simulink model "wlan_mac_hw"  (Simulink 7.8)
settings: Solver=ode45  StartTime=0.0  StopTime=200  RelTol=1e-3
PostLoadFcn:
  | wlan_mac_hw_init
InitFcn:
  | wlan_mac_hw_init
StartFcn:
  | wlan_mac_hw_init
values from neighbouring files (symbols this model uses):
  NB_CNTR_NAV = ceil(log2(MAX_NAV * 160))    [wlan_mac_hw_init.m]
  ticks_per_usec = 10    [wlan_mac_hw_init.m]
undefined symbols (not defined in the file or in its folder): gcbh, xlBlockLoadCallback, xlGetNormalizedPeriod
libraries: xbsIndex_r4 x788, xbsEDKLib_r4 x1
(part 4 of 6)

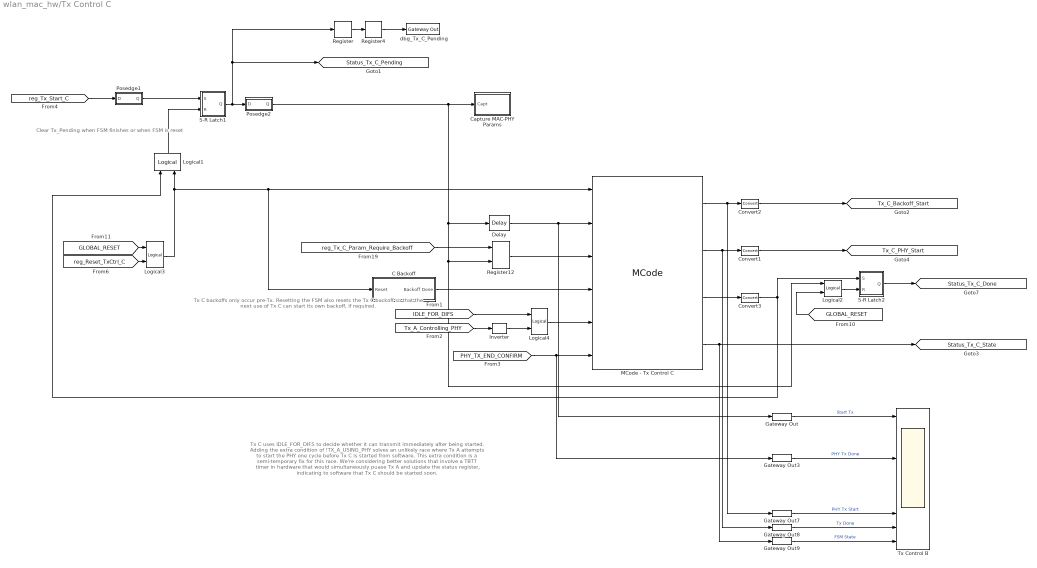
== system wlan_mac_hw/Tx Control C ==
  note: Clear Tx_Pending when FSM finishes
      | or when FSM is reset
  note: Tx C backoffs only occur pre-Tx. Resetting
      | the FSM also resets the Tx C backoff so that
      | the next use of Tx C can start its own backoff,
      | if required.
  note: Tx C uses IDLE_FOR_DIFS to decide whether it can
      | transmit immediately after being started. Adding the
      | extra condition of !TX_A_USING_PHY solves an unlikely
      | race where Tx A attempts to start the PHY one cycle
      | before Tx C is started from software.
      |
      | This extra condition is a semi-temporary fix for this race. We're
      | considering better solutions that involve a TBTT timer in
      | hardware that would simultaneously puase Tx A and update
      | the status register, indicating to software that Tx C should be
      | started soon.
  C Backoff : Subsystem
  Capture MAC-PHY Params : Subsystem
  Convert1 : xbsIndex_r4/Convert  gui_display_data_type=Boolean  arith_type=Boolean  n_bits=16  bin_pt=14  float_type=Single  exp_bits=8  fraction_bits=24  quantization=Truncate  overflow=Wrap  en=off  latency=0  dbl_ovrd=off  pipeline=off  block_type=convert
  Convert2 : xbsIndex_r4/Convert  gui_display_data_type=Boolean  arith_type=Boolean  n_bits=16  bin_pt=14  float_type=Single  exp_bits=8  fraction_bits=24  quantization=Truncate  overflow=Wrap  en=off  latency=0  dbl_ovrd=off  pipeline=off  block_type=convert
  Convert3 : xbsIndex_r4/Convert  gui_display_data_type=Boolean  arith_type=Boolean  n_bits=16  bin_pt=14  float_type=Single  exp_bits=8  fraction_bits=24  quantization=Truncate  overflow=Wrap  en=off  latency=0  dbl_ovrd=off  pipeline=off  block_type=convert
  Delay : xbsIndex_r4/Delay  rst=off  infoeditControl=Selection of Reset will increase slice count due to use of real FFs and instead of SRLs  en=off  latency=1  dbl_ovrd=off  reg_retiming=off  block_type=delay
  Gateway Out{,3,7..9} (5 alike) : xbsIndex_r4/Gateway Out  inherit_from_input=off  hdl_port=off  timing_constraint=None  locs_specified=off  LOCs={}  UseAsDAC=off  DACChannel='1'  block_type=gatewayout
  Inverter : xbsIndex_r4/Inverter  en=off  latency=0  dbl_ovrd=off  block_type=inv
      settings: xl_area=[0 0 0 0 0 0 0]  block_version=VER_STRING_GOES_HERE
  Logical1 : xbsIndex_r4/Logical  logical_function=OR  inputs=2  en=off  latency=0  precision=Full  arith_type=Unsigned  n_bits=8  bin_pt=2  align_bp=on  dbl_ovrd=off  block_type=logical
      settings: xl_area=[1 0 0 1 0 0 0]  block_version=VER_STRING_GOES_HERE
  Logical2 : xbsIndex_r4/Logical  logical_function=OR  inputs=2  en=off  latency=0  precision=Full  arith_type=Unsigned  n_bits=8  bin_pt=2  align_bp=on  dbl_ovrd=off  block_type=logical
      settings: xl_area=[1 0 0 1 0 0 0]  block_version=VER_STRING_GOES_HERE
  Logical3 : xbsIndex_r4/Logical  logical_function=OR  inputs=2  en=off  latency=0  precision=Full  arith_type=Unsigned  n_bits=8  bin_pt=2  align_bp=on  dbl_ovrd=off  block_type=logical
      settings: xl_area=[1 0 0 1 0 0 0]  block_version=VER_STRING_GOES_HERE
  Logical4 : xbsIndex_r4/Logical  logical_function=AND  inputs=2  en=off  latency=0  precision=Full  arith_type=Unsigned  n_bits=8  bin_pt=2  align_bp=on  dbl_ovrd=off  block_type=logical
      settings: xl_area=[1 0 0 1 0 0 0]  block_version=VER_STRING_GOES_HERE
  MCode - Tx Control C : xbsIndex_r4/MCode  mfname=mac_tx_ctrl_c_fsm  explicit_period=on  period=1  inputsTable={'boundInpExpr'=>['','','','',''],'inputs'=>['reset','new_tx','backoff_done','idle_for_difs','phy_tx_done']}  outputsTable={'outputs'=>['backoff_start','phy_tx_start','tx_done','fsm_state_out'],'suppressOut'=>['off','off','off','off']}  dbl_ovrd=off  enable_stdout=off  enable_debug=off  suppress_output=on  defparams={}  hide_port_list={}  block_type=mcode
  Posedge1 : Subsystem
  Posedge2 : Subsystem
  Register : xbsIndex_r4/Register  init=0  rst=off  en=off  dbl_ovrd=off  block_type=register
  Register12 : xbsIndex_r4/Register  init=0  rst=off  en=on  dbl_ovrd=off  block_type=register
  Register4 : xbsIndex_r4/Register  init=0  rst=off  en=off  dbl_ovrd=off  block_type=register
  S-R Latch1 : Subsystem
  S-R Latch2 : Subsystem
  Tx Control B : Scope  NumInputPorts=10
      settings: YMin=-5~-5~-5~-5~-5~-5~-5~-5~-5~-5  YMax=5~5~5~5~5~5~5~5~5~5
  dbg_Tx_C_Pending : xbsIndex_r4/Gateway Out  inherit_from_input=off  hdl_port=on  timing_constraint=None  locs_specified=off  LOCs={}  UseAsDAC=off  DACChannel='1'  block_type=gatewayout
  tag scope: Status_Tx_C_Done=global, Status_Tx_C_Pending=global, Status_Tx_C_State=global, Tx_C_Backoff_Start=global, Tx_C_PHY_Start=global
  wires:
  [reg_Reset_TxCtrl_C] -> Logical3/2
  [GLOBAL_RESET] -> Logical3/1
  Logical3/1 -> Logical1/2, MCode - Tx Control C/1, C Backoff/1(Reset)
  [reg_Tx_Start_C] -> Posedge1/1(D)
  Posedge1/1(Q) -> S-R Latch1/1(S)
  S-R Latch1/1(Q) -> Posedge2/1(D), [Status_Tx_C_Pending], Register/1
  Posedge2/1(Q) -> Capture MAC-PHY Params/1(Capt), Delay/1, Logical2/1, Register12/2
  Delay/1 -> Gateway Out/1, MCode - Tx Control C/2
  [PHY_TX_END_CONFIRM] -> Gateway Out3/1, MCode - Tx Control C/6
  Logical1/1 -> S-R Latch1/2(R)
  MCode - Tx Control C/2 -> Gateway Out8/1, Convert1/1
  MCode - Tx Control C/1 -> Gateway Out7/1, Convert2/1
  MCode - Tx Control C/4 -> [Status_Tx_C_State], Gateway Out9/1
  S-R Latch2/1(Q) -> [Status_Tx_C_Done]
  Convert1/1 -> [Tx_C_PHY_Start]
  Convert3/1 -> Logical1/1, S-R Latch2/1(S)
  Logical2/1 -> S-R Latch2/2(R)
  [GLOBAL_RESET] -> Logical2/2
  Gateway Out/1 -> Tx Control B/1  "Start Tx"
  Gateway Out3/1 -> Tx Control B/4  "PHY Tx Done"
  Gateway Out7/1 -> Tx Control B/8  "PHY Tx Start"
  Gateway Out8/1 -> Tx Control B/9  "Tx Done"
  Gateway Out9/1 -> Tx Control B/10  "FSM State"
  Register/1 -> Register4/1
  Register4/1 -> dbg_Tx_C_Pending/1
  C Backoff/1(Backoff Done) -> MCode - Tx Control C/4
  Logical4/1 -> MCode - Tx Control C/5
  [reg_Tx_C_Param_Require_Backoff] -> Register12/1
  Register12/1 -> MCode - Tx Control C/3
  MCode - Tx Control C/3 -> Convert3/1
  Convert2/1 -> [Tx_C_Backoff_Start]
  [IDLE_FOR_DIFS] -> Logical4/1
  [Tx_A_Controlling_PHY] -> Inverter/1
  Inverter/1 -> Logical4/2

== system wlan_mac_hw/Idle for DIFS-EIFS/Bad Rx ==
  note: Reception with Errors
  Constant1 : xbsIndex_r4/Constant  const=0  gui_display_data_type=Fixed-point  arith_type=Unsigned  n_bits=1  bin_pt=0  preci_type=Single  exp_width=8  frac_width=24  explicit_period=off  period=1  equ=P=C  opselect=C  inp2=PCIN>>17  opr=+  inp1=P  carry=CIN  dbl_ovrd=off  block_type=constant
  Inverter1 : xbsIndex_r4/Inverter  en=off  latency=0  dbl_ovrd=off  block_type=inv
      settings: xl_area=[0 0 0 0 0 0 0]  block_version=VER_STRING_GOES_HERE
  Logical3 : xbsIndex_r4/Logical  logical_function=AND  inputs=2  en=off  latency=0  precision=Full  arith_type=Unsigned  n_bits=16  bin_pt=0  align_bp=on  dbl_ovrd=off  block_type=logical
  Logical4 : xbsIndex_r4/Logical  logical_function=OR  inputs=2  en=off  latency=0  precision=Full  arith_type=Unsigned  n_bits=16  bin_pt=0  align_bp=on  dbl_ovrd=off  block_type=logical
  Posedge1 : Subsystem
  Relational1 : xbsIndex_r4/Relational  mode=a!=b  en=off  latency=0  dbl_ovrd=off  block_type=relational
  Rx : Outport
  wires:
  [PHY_RX_END_IND] -> Logical3/1
  [PHY_RX_FCS_GOOD_IND] -> Inverter1/1
  Inverter1/1 -> Logical4/1
  Logical4/1 -> Logical3/2
  Constant1/1 -> Relational1/2
  [PHY_RX_END_RXERROR] -> Relational1/1
  Relational1/1 -> Logical4/2
  Logical3/1 -> Posedge1/1(D)
  Posedge1/1(Q) -> Rx/1

== system wlan_mac_hw/Idle for DIFS-EIFS/S-R Latch1 ==
  S : Inport
  R : Inport  Port=2
  Constant1 : xbsIndex_r4/Constant  const=1  gui_display_data_type=Boolean  arith_type=Boolean  n_bits=1  bin_pt=0  preci_type=Single  exp_width=8  frac_width=24  explicit_period=off  period=1  equ=P=C  opselect=C  inp2=PCIN>>17  opr=+  inp1=P  carry=CIN  dbl_ovrd=off  block_type=constant
      settings: block_version=VER_STRING_GOES_HERE
  Register2 : xbsIndex_r4/Register  init=0  rst=on  en=on  dbl_ovrd=off  block_type=register
      settings: xl_area=[1 1 0 0 0 0 0]  block_version=VER_STRING_GOES_HERE
  Q : Outport
  wires:
  S/1 -> Register2/3
  Register2/1 -> Q/1
  R/1 -> Register2/2
  Constant1/1 -> Register2/1

== system wlan_mac_hw/NAV/New Duration ==
  note: Only trust DURATION values from
      | packets received with no errors.
      | RX_END_IND always follows last byte
      | and FCS assertion.
      | Skip NAV update on packets addressed
      | to me (handles case of receiving RTS with
      | large DURATION that somehow doesn't lead
      | to CTS/DATA/ACK)
  note: usec
  note: usec/10
  note: clock ticks
  AddSub : xbsIndex_r4/AddSub  mode=Addition  use_carryin=off  use_carryout=off  en=off  latency=0  precision=User Defined  arith_type=Unsigned  n_bits=21  bin_pt=0  quantization=Truncate  overflow=Wrap  dbl_ovrd=off  use_behavioral_HDL=off  hw_selection=Fabric  pipelined=off  block_type=addsub
  Capture Rx Pkt Duration Field : Subsystem
  Check Dest Addr : Subsystem
  Constant1 : xbsIndex_r4/Constant  const=ticks_per_usec  gui_display_data_type=Fixed-point  arith_type=Unsigned  n_bits=ceil(log2(ticks_per_usec))  bin_pt=0  preci_type=Single  exp_width=8  frac_width=24  explicit_period=off  period=1  equ=P=C  opselect=C  inp2=PCIN>>17  opr=+  inp1=P  carry=CIN  dbl_ovrd=off  block_type=constant
  Constant3 : xbsIndex_r4/Constant  const=0  gui_display_data_type=Fixed-point  arith_type=Unsigned  n_bits=1  bin_pt=0  preci_type=Single  exp_width=8  frac_width=24  explicit_period=off  period=1  equ=P=C  opselect=C  inp2=PCIN>>17  opr=+  inp1=P  carry=CIN  dbl_ovrd=off  block_type=constant
  Delay : xbsIndex_r4/Delay  rst=off  infoeditControl=Selection of Reset will increase slice count due to use of real FFs and instead of SRLs  en=off  latency=1  dbl_ovrd=off  reg_retiming=off  block_type=delay
  Delay1 : xbsIndex_r4/Delay  rst=off  infoeditControl=Selection of Reset will increase slice count due to use of real FFs and instead of SRLs  en=off  latency=1  dbl_ovrd=off  reg_retiming=off  block_type=delay
  Inverter : xbsIndex_r4/Inverter  en=off  latency=0  dbl_ovrd=off  block_type=inv
      settings: xl_area=[0 0 0 0 0 0 0]  block_version=VER_STRING_GOES_HERE
  Logical2 : xbsIndex_r4/Logical  logical_function=AND  inputs=4  en=off  latency=0  precision=Full  arith_type=Unsigned  n_bits=16  bin_pt=0  align_bp=on  dbl_ovrd=off  block_type=logical
  Mult : xbsIndex_r4/Mult  precision=Full  arith_type="Signed  (2's comp)"  n_bits=16  bin_pt=14  quantization=Truncate  overflow=Wrap  en=off  latency=1  dbl_ovrd=off  use_behavioral_HDL=off  opt=Speed  use_embedded=on  optimum_pipeline=off  pipeline=on  use_rpm=on  placement_style=Triangular  block_type=mult
  Posedge1 : Subsystem
  Register2 : xbsIndex_r4/Register  init=0  rst=on  en=on  dbl_ovrd=off  block_type=register
  Relational3 : xbsIndex_r4/Relational  mode=a=b  en=off  latency=0  dbl_ovrd=off  block_type=relational
  x16 : Subsystem
  Duration : Outport
  Valid : Outport  Port=2
  wires:
  Capture Rx Pkt Duration Field/1(Duration) -> Register2/1
  Relational3/1 -> Logical2/3
  Constant3/1 -> Relational3/2
  [PHY_RX_END_IND] -> Logical2/2
  [PHY_RX_END_RXERROR] -> Relational3/1
  [Status_Rx_FCS_Good] -> Logical2/1
  Logical2/1 -> Register2/3, Delay/1
  [PHY_RX_START_IND] -> Register2/2
  Register2/1 -> Mult/2
  Delay/1 -> Delay1/1
  Constant1/1 -> Mult/1
  Mult/1 -> AddSub/1
  AddSub/1 -> x16/1(A)
  x16/1(Ax16) -> Duration/1
  Delay1/1 -> Posedge1/1(D)
  Posedge1/1(Q) -> Valid/1
  [reg_NAV_TIME_ADJ] -> AddSub/2
  Check Dest Addr/1(Addr Match) -> Inverter/1
  Inverter/1 -> Logical2/4

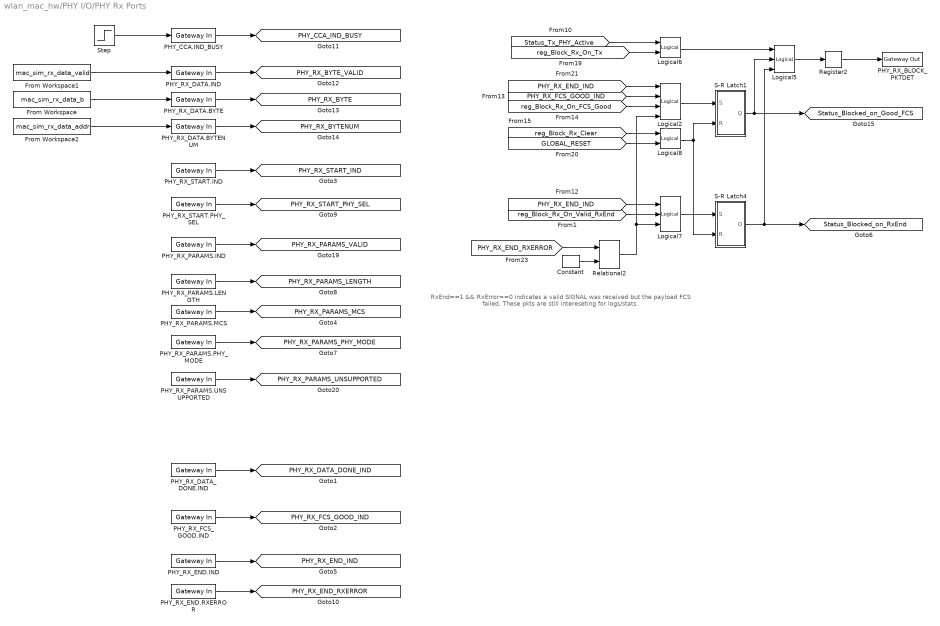
== system wlan_mac_hw/PHY I/O/PHY Rx Ports ==
  note: RxEnd==1 && RxError==0 indicates
      | a valid SIGNAL was received but the payload
      | FCS failed. These pkts are still intereseting
      | for logs/stats.
  Constant : xbsIndex_r4/Constant  const=0  gui_display_data_type=Fixed-point  arith_type=Unsigned  n_bits=1  bin_pt=0  preci_type=Single  exp_width=8  frac_width=24  explicit_period=off  period=1  equ=P=C  opselect=C  inp2=PCIN>>17  opr=+  inp1=P  carry=CIN  dbl_ovrd=off  block_type=constant
  From Workspace : FromWorkspace  VariableName=mac_sim_rx_data_b  SampleTime=1  Interpolate=off  OutputAfterFinalValue=Cyclic repetition
  From Workspace1 : FromWorkspace  VariableName=mac_sim_rx_data_valid  SampleTime=1  Interpolate=off  OutputAfterFinalValue=Cyclic repetition
  From Workspace2 : FromWorkspace  VariableName=mac_sim_rx_data_addr  SampleTime=1  Interpolate=off  OutputAfterFinalValue=Cyclic repetition
  Logical2 : xbsIndex_r4/Logical  logical_function=AND  inputs=4  en=off  latency=0  precision=Full  arith_type=Unsigned  n_bits=8  bin_pt=2  align_bp=on  dbl_ovrd=off  block_type=logical
      settings: xl_area=[1 0 0 1 0 0 0]  block_version=VER_STRING_GOES_HERE
  Logical5 : xbsIndex_r4/Logical  logical_function=OR  inputs=3  en=off  latency=0  precision=Full  arith_type=Unsigned  n_bits=8  bin_pt=2  align_bp=on  dbl_ovrd=off  block_type=logical
      settings: xl_area=[1 0 0 1 0 0 0]  block_version=VER_STRING_GOES_HERE
  Logical6 : xbsIndex_r4/Logical  logical_function=AND  inputs=2  en=off  latency=0  precision=Full  arith_type=Unsigned  n_bits=8  bin_pt=2  align_bp=on  dbl_ovrd=off  block_type=logical
      settings: xl_area=[1 0 0 1 0 0 0]  block_version=VER_STRING_GOES_HERE
  Logical7 : xbsIndex_r4/Logical  logical_function=AND  inputs=3  en=off  latency=0  precision=Full  arith_type=Unsigned  n_bits=8  bin_pt=2  align_bp=on  dbl_ovrd=off  block_type=logical
      settings: xl_area=[1 0 0 1 0 0 0]  block_version=VER_STRING_GOES_HERE
  Logical8 : xbsIndex_r4/Logical  logical_function=OR  inputs=2  en=off  latency=0  precision=Full  arith_type=Unsigned  n_bits=8  bin_pt=2  align_bp=on  dbl_ovrd=off  block_type=logical
      settings: xl_area=[1 0 0 1 0 0 0]  block_version=VER_STRING_GOES_HERE
  PHY_CCA.IND_BUSY : xbsIndex_r4/Gateway In  gui_display_data_type=Boolean  arith_type=Boolean  n_bits=16  bin_pt=14  preci_type=Single  exp_width=8  frac_width=24  quantization="Round  (unbiased: +/- Inf)"  overflow=Saturate  period=1  dbl_ovrd=off  timing_constraint=None  locs_specified=off  LOCs={}  UseAsADC=off  ADCChannel='1'  inherit_from_input=off  hdl_port=on  block_type=gatewayin
  PHY_RX_BLOCK_PKTDET : xbsIndex_r4/Gateway Out  inherit_from_input=off  hdl_port=on  timing_constraint=None  locs_specified=off  LOCs={}  UseAsDAC=off  DACChannel='1'  block_type=gatewayout
  PHY_RX_DATA.BYTE : xbsIndex_r4/Gateway In  gui_display_data_type=Fixed-point  arith_type=Unsigned  n_bits=8  bin_pt=0  preci_type=Single  exp_width=8  frac_width=24  quantization="Round  (unbiased: +/- Inf)"  overflow=Saturate  period=1  dbl_ovrd=off  timing_constraint=None  locs_specified=off  LOCs={}  UseAsADC=off  ADCChannel='1'  inherit_from_input=off  hdl_port=on  block_type=gatewayin
  PHY_RX_DATA.BYTENUM : xbsIndex_r4/Gateway In  gui_display_data_type=Fixed-point  arith_type=Unsigned  n_bits=16  bin_pt=0  preci_type=Single  exp_width=8  frac_width=24  quantization="Round  (unbiased: +/- Inf)"  overflow=Saturate  period=1  dbl_ovrd=off  timing_constraint=None  locs_specified=off  LOCs={}  UseAsADC=off  ADCChannel='1'  inherit_from_input=off  hdl_port=on  block_type=gatewayin
  PHY_RX_DATA.IND : xbsIndex_r4/Gateway In  gui_display_data_type=Boolean  arith_type=Boolean  n_bits=16  bin_pt=14  preci_type=Single  exp_width=8  frac_width=24  quantization="Round  (unbiased: +/- Inf)"  overflow=Saturate  period=1  dbl_ovrd=off  timing_constraint=None  locs_specified=off  LOCs={}  UseAsADC=off  ADCChannel='1'  inherit_from_input=off  hdl_port=on  block_type=gatewayin
  PHY_RX_DATA_DONE.IND : xbsIndex_r4/Gateway In  gui_display_data_type=Boolean  arith_type=Boolean  n_bits=1  bin_pt=0  preci_type=Single  exp_width=8  frac_width=24  quantization="Round  (unbiased: +/- Inf)"  overflow=Saturate  period=1  dbl_ovrd=off  timing_constraint=None  locs_specified=off  LOCs={}  UseAsADC=off  ADCChannel='1'  inherit_from_input=off  hdl_port=on  block_type=gatewayin
  PHY_RX_END.IND : xbsIndex_r4/Gateway In  gui_display_data_type=Boolean  arith_type=Boolean  n_bits=16  bin_pt=14  preci_type=Single  exp_width=8  frac_width=24  quantization="Round  (unbiased: +/- Inf)"  overflow=Saturate  period=1  dbl_ovrd=off  timing_constraint=None  locs_specified=off  LOCs={}  UseAsADC=off  ADCChannel='1'  inherit_from_input=off  hdl_port=on  block_type=gatewayin
  PHY_RX_END.RXERROR : xbsIndex_r4/Gateway In  gui_display_data_type=Fixed-point  arith_type=Unsigned  n_bits=4  bin_pt=0  preci_type=Single  exp_width=8  frac_width=24  quantization="Round  (unbiased: +/- Inf)"  overflow=Saturate  period=1  dbl_ovrd=off  timing_constraint=None  locs_specified=off  LOCs={}  UseAsADC=off  ADCChannel='1'  inherit_from_input=off  hdl_port=on  block_type=gatewayin
  PHY_RX_FCS_GOOD.IND : xbsIndex_r4/Gateway In  gui_display_data_type=Boolean  arith_type=Boolean  n_bits=1  bin_pt=0  preci_type=Single  exp_width=8  frac_width=24  quantization="Round  (unbiased: +/- Inf)"  overflow=Saturate  period=1  dbl_ovrd=off  timing_constraint=None  locs_specified=off  LOCs={}  UseAsADC=off  ADCChannel='1'  inherit_from_input=off  hdl_port=on  block_type=gatewayin
  PHY_RX_PARAMS.IND : xbsIndex_r4/Gateway In  gui_display_data_type=Boolean  arith_type=Boolean  n_bits=16  bin_pt=14  preci_type=Single  exp_width=8  frac_width=24  quantization="Round  (unbiased: +/- Inf)"  overflow=Saturate  period=1  dbl_ovrd=off  timing_constraint=None  locs_specified=off  LOCs={}  UseAsADC=off  ADCChannel='1'  inherit_from_input=off  hdl_port=on  block_type=gatewayin
  PHY_RX_PARAMS.LENGTH : xbsIndex_r4/Gateway In  gui_display_data_type=Fixed-point  arith_type=Unsigned  n_bits=16  bin_pt=0  preci_type=Single  exp_width=8  frac_width=24  quantization="Round  (unbiased: +/- Inf)"  overflow=Saturate  period=1  dbl_ovrd=off  timing_constraint=None  locs_specified=off  LOCs={}  UseAsADC=off  ADCChannel='1'  inherit_from_input=off  hdl_port=on  block_type=gatewayin
  PHY_RX_PARAMS.MCS : xbsIndex_r4/Gateway In  gui_display_data_type=Fixed-point  arith_type=Unsigned  n_bits=7  bin_pt=0  preci_type=Single  exp_width=8  frac_width=24  quantization="Round  (unbiased: +/- Inf)"  overflow=Saturate  period=1  dbl_ovrd=off  timing_constraint=None  locs_specified=off  LOCs={}  UseAsADC=off  ADCChannel='1'  inherit_from_input=off  hdl_port=on  block_type=gatewayin
  PHY_RX_PARAMS.PHY_MODE : xbsIndex_r4/Gateway In  gui_display_data_type=Fixed-point  arith_type=Unsigned  n_bits=3  bin_pt=0  preci_type=Single  exp_width=8  frac_width=24  quantization="Round  (unbiased: +/- Inf)"  overflow=Saturate  period=1  dbl_ovrd=off  timing_constraint=None  locs_specified=off  LOCs={}  UseAsADC=off  ADCChannel='1'  inherit_from_input=off  hdl_port=on  block_type=gatewayin
  PHY_RX_PARAMS.UNSUPPORTED : xbsIndex_r4/Gateway In  gui_display_data_type=Boolean  arith_type=Boolean  n_bits=16  bin_pt=14  preci_type=Single  exp_width=8  frac_width=24  quantization="Round  (unbiased: +/- Inf)"  overflow=Saturate  period=1  dbl_ovrd=off  timing_constraint=None  locs_specified=off  LOCs={}  UseAsADC=off  ADCChannel='1'  inherit_from_input=off  hdl_port=on  block_type=gatewayin
  PHY_RX_START.IND : xbsIndex_r4/Gateway In  gui_display_data_type=Boolean  arith_type=Boolean  n_bits=16  bin_pt=14  preci_type=Single  exp_width=8  frac_width=24  quantization="Round  (unbiased: +/- Inf)"  overflow=Saturate  period=1  dbl_ovrd=off  timing_constraint=None  locs_specified=off  LOCs={}  UseAsADC=off  ADCChannel='1'  inherit_from_input=off  hdl_port=on  block_type=gatewayin
  PHY_RX_START.PHY_SEL : xbsIndex_r4/Gateway In  gui_display_data_type=Boolean  arith_type=Boolean  n_bits=16  bin_pt=14  preci_type=Single  exp_width=8  frac_width=24  quantization="Round  (unbiased: +/- Inf)"  overflow=Saturate  period=1  dbl_ovrd=off  timing_constraint=None  locs_specified=off  LOCs={}  UseAsADC=off  ADCChannel='1'  inherit_from_input=off  hdl_port=on  block_type=gatewayin
  Register2 : xbsIndex_r4/Register  init=0  rst=off  en=off  dbl_ovrd=off  block_type=register
  Relational2 : xbsIndex_r4/Relational  mode=a=b  en=off  latency=0  dbl_ovrd=off  block_type=relational
  S-R Latch1 : Subsystem
  S-R Latch4 : Subsystem
  Step : Step  Time=6e3  Before=1  After=0  SampleTime=1
  tag scope: PHY_CCA_IND_BUSY=global, PHY_RX_BYTE=global, PHY_RX_BYTENUM=global, PHY_RX_BYTE_VALID=global, PHY_RX_DATA_DONE_IND=global, PHY_RX_END_IND=global, PHY_RX_END_RXERROR=global, PHY_RX_FCS_GOOD_IND=global, PHY_RX_PARAMS_LENGTH=global, PHY_RX_PARAMS_MCS=global, PHY_RX_PARAMS_PHY_MODE=global, PHY_RX_PARAMS_UNSUPPORTED=global, PHY_RX_PARAMS_VALID=global, PHY_RX_START_IND=global, PHY_RX_START_PHY_SEL=global, Status_Blocked_on_Good_FCS=global, Status_Blocked_on_RxEnd=global
  wires:
  PHY_RX_DATA_DONE.IND/1 -> [PHY_RX_DATA_DONE_IND]
  PHY_RX_FCS_GOOD.IND/1 -> [PHY_RX_FCS_GOOD_IND]
  PHY_RX_START.IND/1 -> [PHY_RX_START_IND]
  PHY_RX_PARAMS.MCS/1 -> [PHY_RX_PARAMS_MCS]
  PHY_RX_END.IND/1 -> [PHY_RX_END_IND]
  PHY_RX_END.RXERROR/1 -> [PHY_RX_END_RXERROR]
  PHY_CCA.IND_BUSY/1 -> [PHY_CCA_IND_BUSY]
  PHY_RX_DATA.IND/1 -> [PHY_RX_BYTE_VALID]
  PHY_RX_DATA.BYTE/1 -> [PHY_RX_BYTE]
  PHY_RX_DATA.BYTENUM/1 -> [PHY_RX_BYTENUM]
  PHY_RX_START.PHY_SEL/1 -> [PHY_RX_START_PHY_SEL]
  Step/1 -> PHY_CCA.IND_BUSY/1
  PHY_RX_PARAMS.LENGTH/1 -> [PHY_RX_PARAMS_LENGTH]
  PHY_RX_PARAMS.IND/1 -> [PHY_RX_PARAMS_VALID]
  PHY_RX_PARAMS.PHY_MODE/1 -> [PHY_RX_PARAMS_PHY_MODE]
  PHY_RX_PARAMS.UNSUPPORTED/1 -> [PHY_RX_PARAMS_UNSUPPORTED]
  Register2/1 -> PHY_RX_BLOCK_PKTDET/1
  Logical6/1 -> Logical5/1
  S-R Latch1/1(Q) -> Logical5/2, [Status_Blocked_on_Good_FCS]
  Logical5/1 -> Register2/1
  Logical8/1 -> S-R Latch1/2(R), S-R Latch4/2(R)
  [reg_Block_Rx_Clear] -> Logical8/1
  [GLOBAL_RESET] -> Logical8/2
  [Status_Tx_PHY_Active] -> Logical6/1
  [reg_Block_Rx_On_Tx] -> Logical6/2
  Logical2/1 -> S-R Latch1/1(S)
  S-R Latch4/1(Q) -> Logical5/3, [Status_Blocked_on_RxEnd]
  Logical7/1 -> S-R Latch4/1(S)
  [PHY_RX_END_IND] -> Logical7/1
  Constant/1 -> Relational2/2
  [PHY_RX_END_RXERROR] -> Relational2/1
  [reg_Block_Rx_On_Valid_RxEnd] -> Logical7/2
  Relational2/1 -> Logical7/3, Logical2/4
  [PHY_RX_END_IND] -> Logical2/1
  [PHY_RX_FCS_GOOD_IND] -> Logical2/2
  [reg_Block_Rx_On_FCS_Good] -> Logical2/3
  From Workspace/1 -> PHY_RX_DATA.BYTE/1
  From Workspace1/1 -> PHY_RX_DATA.IND/1
  From Workspace2/1 -> PHY_RX_DATA.BYTENUM/1

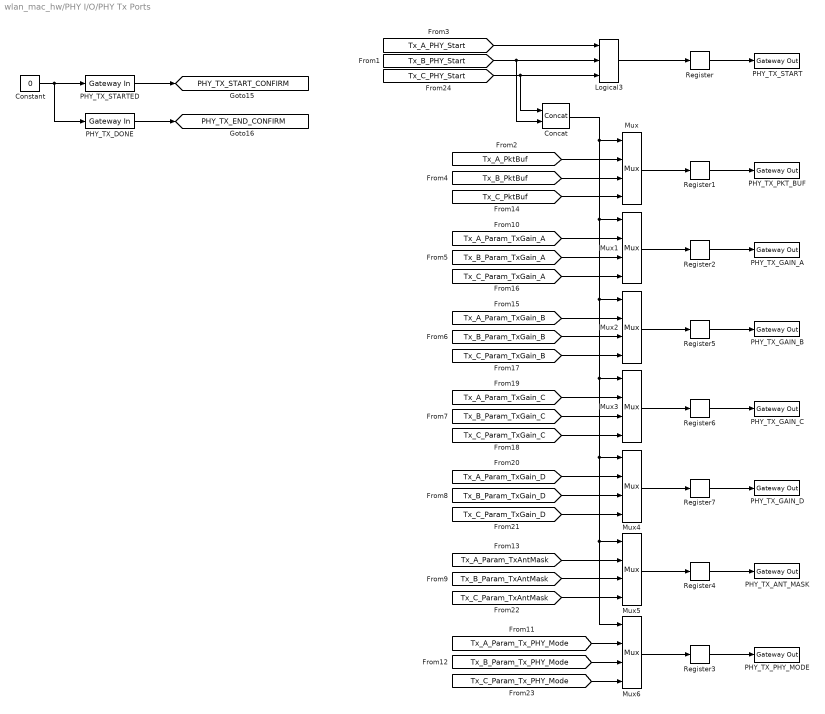
== system wlan_mac_hw/PHY I/O/PHY Tx Ports ==
  Concat : xbsIndex_r4/Concat  num_inputs=2  dbl_ovrd=off  block_type=concat
  Constant : Constant  Value=0
  Logical3 : xbsIndex_r4/Logical  logical_function=OR  inputs=3  en=off  latency=0  precision=Full  arith_type=Unsigned  n_bits=16  bin_pt=0  align_bp=on  dbl_ovrd=off  block_type=logical
  Mux{,1..6} (7 alike) : xbsIndex_r4/Mux  inputs=3  en=off  latency=0  precision=Full  arith_type=Unsigned  n_bits=16  bin_pt=14  quantization=Truncate  overflow=Wrap  dbl_ovrd=off  block_type=mux
  PHY_TX_ANT_MASK : xbsIndex_r4/Gateway Out  inherit_from_input=off  hdl_port=on  timing_constraint=None  locs_specified=off  LOCs={}  UseAsDAC=off  DACChannel='1'  block_type=gatewayout
  PHY_TX_DONE : xbsIndex_r4/Gateway In  gui_display_data_type=Boolean  arith_type=Boolean  n_bits=16  bin_pt=14  preci_type=Single  exp_width=8  frac_width=24  quantization="Round  (unbiased: +/- Inf)"  overflow=Saturate  period=1  dbl_ovrd=off  timing_constraint=None  locs_specified=off  LOCs={}  UseAsADC=off  ADCChannel='1'  inherit_from_input=off  hdl_port=on  block_type=gatewayin
  PHY_TX_GAIN_A : xbsIndex_r4/Gateway Out  inherit_from_input=off  hdl_port=on  timing_constraint=None  locs_specified=off  LOCs={}  UseAsDAC=off  DACChannel='1'  block_type=gatewayout
  PHY_TX_GAIN_B : xbsIndex_r4/Gateway Out  inherit_from_input=off  hdl_port=on  timing_constraint=None  locs_specified=off  LOCs={}  UseAsDAC=off  DACChannel='1'  block_type=gatewayout
  PHY_TX_GAIN_C : xbsIndex_r4/Gateway Out  inherit_from_input=off  hdl_port=on  timing_constraint=None  locs_specified=off  LOCs={}  UseAsDAC=off  DACChannel='1'  block_type=gatewayout
  PHY_TX_GAIN_D : xbsIndex_r4/Gateway Out  inherit_from_input=off  hdl_port=on  timing_constraint=None  locs_specified=off  LOCs={}  UseAsDAC=off  DACChannel='1'  block_type=gatewayout
  PHY_TX_PHY_MODE : xbsIndex_r4/Gateway Out  inherit_from_input=off  hdl_port=on  timing_constraint=None  locs_specified=off  LOCs={}  UseAsDAC=off  DACChannel='1'  block_type=gatewayout
  PHY_TX_PKT_BUF : xbsIndex_r4/Gateway Out  inherit_from_input=off  hdl_port=on  timing_constraint=None  locs_specified=off  LOCs={}  UseAsDAC=off  DACChannel='1'  block_type=gatewayout
  PHY_TX_START : xbsIndex_r4/Gateway Out  inherit_from_input=off  hdl_port=on  timing_constraint=None  locs_specified=off  LOCs={}  UseAsDAC=off  DACChannel='1'  block_type=gatewayout
  PHY_TX_STARTED : xbsIndex_r4/Gateway In  gui_display_data_type=Boolean  arith_type=Boolean  n_bits=16  bin_pt=14  preci_type=Single  exp_width=8  frac_width=24  quantization="Round  (unbiased: +/- Inf)"  overflow=Saturate  period=1  dbl_ovrd=off  timing_constraint=None  locs_specified=off  LOCs={}  UseAsADC=off  ADCChannel='1'  inherit_from_input=off  hdl_port=on  block_type=gatewayin
  Register{,1..7} (8 alike) : xbsIndex_r4/Register  init=0  rst=off  en=off  dbl_ovrd=off  block_type=register
  tag scope: PHY_TX_END_CONFIRM=global, PHY_TX_START_CONFIRM=global
  wires:
  Register7/1 -> PHY_TX_GAIN_D/1
  Register6/1 -> PHY_TX_GAIN_C/1
  Register5/1 -> PHY_TX_GAIN_B/1
  Register4/1 -> PHY_TX_ANT_MASK/1
  Register2/1 -> PHY_TX_GAIN_A/1
  Register1/1 -> PHY_TX_PKT_BUF/1
  Register/1 -> PHY_TX_START/1
  Mux/1 -> Register1/1
  Concat/1 -> Mux/1, Mux1/1, Mux2/1, Mux3/1, Mux4/1, Mux5/1, Mux6/1
  PHY_TX_DONE/1 -> [PHY_TX_END_CONFIRM]
  PHY_TX_STARTED/1 -> [PHY_TX_START_CONFIRM]
  Constant/1 -> PHY_TX_STARTED/1, PHY_TX_DONE/1
  Register3/1 -> PHY_TX_PHY_MODE/1
  [Tx_A_PktBuf] -> Mux/2
  [Tx_B_PktBuf] -> Mux/3
  [Tx_C_PktBuf] -> Mux/4
  [Tx_A_Param_TxGain_A] -> Mux1/2
  [Tx_B_Param_TxGain_A] -> Mux1/3
  [Tx_C_Param_TxGain_A] -> Mux1/4
  [Tx_A_Param_TxGain_B] -> Mux2/2
  [Tx_B_Param_TxGain_B] -> Mux2/3
  [Tx_C_Param_TxGain_B] -> Mux2/4
  [Tx_A_Param_TxGain_C] -> Mux3/2
  [Tx_B_Param_TxGain_C] -> Mux3/3
  [Tx_C_Param_TxGain_C] -> Mux3/4
  [Tx_A_Param_TxGain_D] -> Mux4/2
  [Tx_B_Param_TxGain_D] -> Mux4/3
  [Tx_C_Param_TxGain_D] -> Mux4/4
  [Tx_A_Param_TxAntMask] -> Mux5/2
  [Tx_B_Param_TxAntMask] -> Mux5/3
  [Tx_C_Param_TxAntMask] -> Mux5/4
  [Tx_A_Param_Tx_PHY_Mode] -> Mux6/2
  [Tx_B_Param_Tx_PHY_Mode] -> Mux6/3
  [Tx_C_Param_Tx_PHY_Mode] -> Mux6/4
  Mux6/1 -> Register3/1
  Mux5/1 -> Register4/1
  Mux4/1 -> Register7/1
  Mux3/1 -> Register6/1
  Mux2/1 -> Register5/1
  Mux1/1 -> Register2/1
  [Tx_A_PHY_Start] -> Logical3/1
  [Tx_B_PHY_Start] -> Logical3/2, Concat/2
  [Tx_C_PHY_Start] -> Logical3/3, Concat/1
  Logical3/1 -> Register/1

== system wlan_mac_hw/PHY I/O/S-R Latch2 ==
  S : Inport
  R : Inport  Port=2
  Constant1 : xbsIndex_r4/Constant  const=1  gui_display_data_type=Boolean  arith_type=Boolean  n_bits=1  bin_pt=0  preci_type=Single  exp_width=8  frac_width=24  explicit_period=off  period=1  equ=P=C  opselect=C  inp2=PCIN>>17  opr=+  inp1=P  carry=CIN  dbl_ovrd=off  block_type=constant
      settings: block_version=VER_STRING_GOES_HERE
  Register2 : xbsIndex_r4/Register  init=0  rst=on  en=on  dbl_ovrd=off  block_type=register
      settings: xl_area=[1 1 0 0 0 0 0]  block_version=VER_STRING_GOES_HERE
  Q : Outport
  wires:
  Constant1/1 -> Register2/1
  R/1 -> Register2/2
  Register2/1 -> Q/1
  S/1 -> Register2/3

== system wlan_mac_hw/PHY I/O/S-R Latch3 ==
  S : Inport
  R : Inport  Port=2
  Constant1 : xbsIndex_r4/Constant  const=1  gui_display_data_type=Boolean  arith_type=Boolean  n_bits=1  bin_pt=0  preci_type=Single  exp_width=8  frac_width=24  explicit_period=off  period=1  equ=P=C  opselect=C  inp2=PCIN>>17  opr=+  inp1=P  carry=CIN  dbl_ovrd=off  block_type=constant
      settings: block_version=VER_STRING_GOES_HERE
  Register2 : xbsIndex_r4/Register  init=0  rst=on  en=on  dbl_ovrd=off  block_type=register
      settings: xl_area=[1 1 0 0 0 0 0]  block_version=VER_STRING_GOES_HERE
  Q : Outport
  wires:
  S/1 -> Register2/3
  Register2/1 -> Q/1
  R/1 -> Register2/2
  Constant1/1 -> Register2/1

== system wlan_mac_hw/Post Tx/Rx Timers/Posedge1 ==
  note: Rising Edge Detection
  D : Inport
  Delay : xbsIndex_r4/Delay  rst=off  infoeditControl=Selection of Reset will increase slice count due to use of real FFs and instead of SRLs  en=off  latency=1  dbl_ovrd=off  reg_retiming=off  block_type=delay
      settings: infoedit=Hardware notes: A delay line is a chain, each link of which is an SRL16 followed by a flip-flop. If register retiming is enabled, the delay line is a chain of flip-flops.  xl_area=[1 1 0 0 0 0 0]  block_version=VER_STRING_GOES_HERE
  Inverter : xbsIndex_r4/Inverter  en=off  latency=0  dbl_ovrd=off  block_type=inv
      settings: xl_area=[0 0 0 0 0 0 0]  block_version=VER_STRING_GOES_HERE
  Logical1 : xbsIndex_r4/Logical  logical_function=AND  inputs=2  en=off  latency=0  precision=Full  arith_type=Unsigned  n_bits=8  bin_pt=2  align_bp=on  dbl_ovrd=off  block_type=logical
      settings: xl_area=[1 0 0 1 0 0 0]  block_version=VER_STRING_GOES_HERE
  Q : Outport
  wires:
  D/1 -> Logical1/2, Delay/1
  Logical1/1 -> Q/1
  Inverter/1 -> Logical1/1
  Delay/1 -> Inverter/1

== system wlan_mac_hw/Post Tx/Rx Timers/Posedge3 ==
  note: Rising Edge Detection
  D : Inport
  Delay : xbsIndex_r4/Delay  rst=off  infoeditControl=Selection of Reset will increase slice count due to use of real FFs and instead of SRLs  en=off  latency=1  dbl_ovrd=off  reg_retiming=off  block_type=delay
      settings: infoedit=Hardware notes: A delay line is a chain, each link of which is an SRL16 followed by a flip-flop. If register retiming is enabled, the delay line is a chain of flip-flops.  xl_area=[1 1 0 0 0 0 0]  block_version=VER_STRING_GOES_HERE
  Inverter : xbsIndex_r4/Inverter  en=off  latency=0  dbl_ovrd=off  block_type=inv
      settings: xl_area=[0 0 0 0 0 0 0]  block_version=VER_STRING_GOES_HERE
  Logical1 : xbsIndex_r4/Logical  logical_function=AND  inputs=2  en=off  latency=0  precision=Full  arith_type=Unsigned  n_bits=8  bin_pt=2  align_bp=on  dbl_ovrd=off  block_type=logical
      settings: xl_area=[1 0 0 1 0 0 0]  block_version=VER_STRING_GOES_HERE
  Q : Outport
  wires:
  Delay/1 -> Inverter/1
  Inverter/1 -> Logical1/1
  Logical1/1 -> Q/1
  D/1 -> Delay/1, Logical1/2

== system wlan_mac_hw/Post Tx/Rx Timers/S-R Latch1 ==
  S : Inport
  R : Inport  Port=2
  Constant1 : xbsIndex_r4/Constant  const=1  gui_display_data_type=Boolean  arith_type=Boolean  n_bits=1  bin_pt=0  preci_type=Single  exp_width=8  frac_width=24  explicit_period=off  period=1  equ=P=C  opselect=C  inp2=PCIN>>17  opr=+  inp1=P  carry=CIN  dbl_ovrd=off  block_type=constant
      settings: block_version=VER_STRING_GOES_HERE
  Register2 : xbsIndex_r4/Register  init=0  rst=on  en=on  dbl_ovrd=off  block_type=register
      settings: xl_area=[1 1 0 0 0 0 0]  block_version=VER_STRING_GOES_HERE
  Q : Outport
  wires:
  Constant1/1 -> Register2/1
  R/1 -> Register2/2
  Register2/1 -> Q/1
  S/1 -> Register2/3

== system wlan_mac_hw/Post Tx/Rx Timers/S-R Latch2 ==
  S : Inport
  R : Inport  Port=2
  Constant1 : xbsIndex_r4/Constant  const=1  gui_display_data_type=Boolean  arith_type=Boolean  n_bits=1  bin_pt=0  preci_type=Single  exp_width=8  frac_width=24  explicit_period=off  period=1  equ=P=C  opselect=C  inp2=PCIN>>17  opr=+  inp1=P  carry=CIN  dbl_ovrd=off  block_type=constant
      settings: block_version=VER_STRING_GOES_HERE
  Register2 : xbsIndex_r4/Register  init=0  rst=on  en=on  dbl_ovrd=off  block_type=register
      settings: xl_area=[1 1 0 0 0 0 0]  block_version=VER_STRING_GOES_HERE
  Q : Outport
  wires:
  S/1 -> Register2/3
  Register2/1 -> Q/1
  R/1 -> Register2/2
  Constant1/1 -> Register2/1

== system wlan_mac_hw/Post Tx/Rx Timers/S-R Latch3 ==
  S : Inport
  R : Inport  Port=2
  Constant1 : xbsIndex_r4/Constant  const=1  gui_display_data_type=Boolean  arith_type=Boolean  n_bits=1  bin_pt=0  preci_type=Single  exp_width=8  frac_width=24  explicit_period=off  period=1  equ=P=C  opselect=C  inp2=PCIN>>17  opr=+  inp1=P  carry=CIN  dbl_ovrd=off  block_type=constant
      settings: block_version=VER_STRING_GOES_HERE
  Register2 : xbsIndex_r4/Register  init=0  rst=on  en=on  dbl_ovrd=off  block_type=register
      settings: xl_area=[1 1 0 0 0 0 0]  block_version=VER_STRING_GOES_HERE
  Q : Outport
  wires:
  S/1 -> Register2/3
  Register2/1 -> Q/1
  R/1 -> Register2/2
  Constant1/1 -> Register2/1

== system wlan_mac_hw/Post Tx/Rx Timers/S-R Latch4 ==
  S : Inport
  R : Inport  Port=2
  Constant1 : xbsIndex_r4/Constant  const=1  gui_display_data_type=Boolean  arith_type=Boolean  n_bits=1  bin_pt=0  preci_type=Single  exp_width=8  frac_width=24  explicit_period=off  period=1  equ=P=C  opselect=C  inp2=PCIN>>17  opr=+  inp1=P  carry=CIN  dbl_ovrd=off  block_type=constant
      settings: block_version=VER_STRING_GOES_HERE
  Register2 : xbsIndex_r4/Register  init=0  rst=on  en=on  dbl_ovrd=off  block_type=register
      settings: xl_area=[1 1 0 0 0 0 0]  block_version=VER_STRING_GOES_HERE
  Q : Outport
  wires:
  Constant1/1 -> Register2/1
  R/1 -> Register2/2
  Register2/1 -> Q/1
  S/1 -> Register2/3

== system wlan_mac_hw/Registers/Ctrl Bits ==
  32b : Inport
  Posedge1 : Subsystem
  Sim Reset : Subsystem
  b[0] : xbsIndex_r4/Slice  nbits=1  boolean_output=on  mode=Lower Bit Location + Width  bit1=0  base1=MSB of Input  bit0=0  base0=LSB of Input  dbl_ovrd=off  block_type=slice
      settings: block_version=VER_STRING_GOES_HERE
  b[10] : xbsIndex_r4/Slice  nbits=1  boolean_output=on  mode=Lower Bit Location + Width  bit1=0  base1=MSB of Input  bit0=10  base0=LSB of Input  dbl_ovrd=off  block_type=slice
      settings: block_version=VER_STRING_GOES_HERE
  b[11] : xbsIndex_r4/Slice  nbits=1  boolean_output=on  mode=Lower Bit Location + Width  bit1=0  base1=MSB of Input  bit0=11  base0=LSB of Input  dbl_ovrd=off  block_type=slice
      settings: block_version=VER_STRING_GOES_HERE
  b[12] : xbsIndex_r4/Slice  nbits=1  boolean_output=on  mode=Lower Bit Location + Width  bit1=0  base1=MSB of Input  bit0=12  base0=LSB of Input  dbl_ovrd=off  block_type=slice
      settings: block_version=VER_STRING_GOES_HERE
  b[13] : xbsIndex_r4/Slice  nbits=1  boolean_output=on  mode=Lower Bit Location + Width  bit1=0  base1=MSB of Input  bit0=13  base0=LSB of Input  dbl_ovrd=off  block_type=slice
      settings: block_version=VER_STRING_GOES_HERE
  b[14] : xbsIndex_r4/Slice  nbits=1  boolean_output=on  mode=Lower Bit Location + Width  bit1=0  base1=MSB of Input  bit0=14  base0=LSB of Input  dbl_ovrd=off  block_type=slice
      settings: block_version=VER_STRING_GOES_HERE
  b[15] : xbsIndex_r4/Slice  nbits=1  boolean_output=on  mode=Lower Bit Location + Width  bit1=0  base1=MSB of Input  bit0=15  base0=LSB of Input  dbl_ovrd=off  block_type=slice
      settings: block_version=VER_STRING_GOES_HERE
  b[16] : xbsIndex_r4/Slice  nbits=1  boolean_output=on  mode=Lower Bit Location + Width  bit1=0  base1=MSB of Input  bit0=16  base0=LSB of Input  dbl_ovrd=off  block_type=slice
      settings: block_version=VER_STRING_GOES_HERE
  b[17] : xbsIndex_r4/Slice  nbits=1  boolean_output=on  mode=Lower Bit Location + Width  bit1=0  base1=MSB of Input  bit0=17  base0=LSB of Input  dbl_ovrd=off  block_type=slice
      settings: block_version=VER_STRING_GOES_HERE
  "b[1]  " : xbsIndex_r4/Slice  nbits=1  boolean_output=on  mode=Lower Bit Location + Width  bit1=0  base1=MSB of Input  bit0=1  base0=LSB of Input  dbl_ovrd=off  block_type=slice
      settings: block_version=VER_STRING_GOES_HERE
  b[2] : xbsIndex_r4/Slice  nbits=1  boolean_output=on  mode=Lower Bit Location + Width  bit1=0  base1=MSB of Input  bit0=2  base0=LSB of Input  dbl_ovrd=off  block_type=slice
      settings: block_version=VER_STRING_GOES_HERE
  b[3] : xbsIndex_r4/Slice  nbits=1  boolean_output=on  mode=Lower Bit Location + Width  bit1=0  base1=MSB of Input  bit0=3  base0=LSB of Input  dbl_ovrd=off  block_type=slice
      settings: block_version=VER_STRING_GOES_HERE
  b[4] : xbsIndex_r4/Slice  nbits=1  boolean_output=on  mode=Lower Bit Location + Width  bit1=0  base1=MSB of Input  bit0=4  base0=LSB of Input  dbl_ovrd=off  block_type=slice
      settings: block_version=VER_STRING_GOES_HERE
  b[5] : xbsIndex_r4/Slice  nbits=1  boolean_output=on  mode=Lower Bit Location + Width  bit1=0  base1=MSB of Input  bit0=5  base0=LSB of Input  dbl_ovrd=off  block_type=slice
      settings: block_version=VER_STRING_GOES_HERE
  b[6] : xbsIndex_r4/Slice  nbits=1  boolean_output=on  mode=Lower Bit Location + Width  bit1=0  base1=MSB of Input  bit0=6  base0=LSB of Input  dbl_ovrd=off  block_type=slice
      settings: block_version=VER_STRING_GOES_HERE
  b[7] : xbsIndex_r4/Slice  nbits=1  boolean_output=on  mode=Lower Bit Location + Width  bit1=0  base1=MSB of Input  bit0=7  base0=LSB of Input  dbl_ovrd=off  block_type=slice
      settings: block_version=VER_STRING_GOES_HERE
  b[8] : xbsIndex_r4/Slice  nbits=1  boolean_output=on  mode=Lower Bit Location + Width  bit1=0  base1=MSB of Input  bit0=8  base0=LSB of Input  dbl_ovrd=off  block_type=slice
      settings: block_version=VER_STRING_GOES_HERE
  b[9] : xbsIndex_r4/Slice  nbits=1  boolean_output=on  mode=Lower Bit Location + Width  bit1=0  base1=MSB of Input  bit0=9  base0=LSB of Input  dbl_ovrd=off  block_type=slice
      settings: block_version=VER_STRING_GOES_HERE
  tag scope: GLOBAL_RESET=global, reg_Block_Rx_Clear=global, reg_Block_Rx_On_FCS_Good=global, reg_Block_Rx_On_Tx=global, reg_Block_Rx_On_Valid_RxEnd=global, reg_CCA_Force_Busy=global, reg_CCA_Ignore_NAV=global, reg_CCA_Ignore_PHY_CS=global, reg_CCA_Ignore_TxBusy=global, reg_Disable_NAV=global, reg_Force_Reset_A_Backoff=global, reg_Force_Reset_C_Backoff=global, reg_Force_Reset_NAV=global, reg_Pause_A_Backoff=global, reg_Reset_TU_Latch=global, reg_Reset_TxCtrl_A=global, reg_Reset_TxCtrl_B=global, reg_Reset_TxCtrl_C=global
  wires:
  b[0]/1 -> [GLOBAL_RESET]
  32b/1 -> b[0]/1, "b[1]  "/1, b[2]/1, b[3]/1, b[4]/1, b[5]/1, b[6]/1, b[7]/1, b[8]/1, b[9]/1, b[10]/1, b[11]/1, b[12]/1, b[13]/1, b[14]/1, b[15]/1, b[16]/1, b[17]/1
  "b[1]  "/1 -> [reg_Block_Rx_On_FCS_Good]
  b[2]/1 -> Posedge1/1(D)
  Posedge1/1(Q) -> [reg_Block_Rx_Clear]
  b[3]/1 -> [reg_Disable_NAV]
  b[4]/1 -> [reg_Block_Rx_On_Tx]
  b[6]/1 -> [reg_Block_Rx_On_Valid_RxEnd]
  b[7]/1 -> [reg_CCA_Ignore_PHY_CS]
  b[8]/1 -> [reg_CCA_Ignore_TxBusy]
  b[9]/1 -> [reg_CCA_Ignore_NAV]
  b[10]/1 -> [reg_Force_Reset_NAV]
  b[11]/1 -> [reg_Force_Reset_A_Backoff]
  b[12]/1 -> [reg_Force_Reset_C_Backoff]
  b[13]/1 -> [reg_Reset_TxCtrl_A]
  b[14]/1 -> [reg_Reset_TxCtrl_B]
  b[15]/1 -> [reg_Reset_TxCtrl_C]
  b[16]/1 -> [reg_CCA_Force_Busy]
  b[17]/1 -> [reg_Pause_A_Backoff]
  b[5]/1 -> [reg_Reset_TU_Latch]

== system wlan_mac_hw/Registers/Posedge3 ==
  note: Rising Edge Detection
  D : Inport
  Delay : xbsIndex_r4/Delay  rst=off  infoeditControl=Selection of Reset will increase slice count due to use of real FFs and instead of SRLs  en=off  latency=1  dbl_ovrd=off  reg_retiming=off  block_type=delay
      settings: infoedit=Hardware notes: A delay line is a chain, each link of which is an SRL16 followed by a flip-flop. If register retiming is enabled, the delay line is a chain of flip-flops.  xl_area=[1 1 0 0 0 0 0]  block_version=VER_STRING_GOES_HERE
  Inverter : xbsIndex_r4/Inverter  en=off  latency=0  dbl_ovrd=off  block_type=inv
      settings: xl_area=[0 0 0 0 0 0 0]  block_version=VER_STRING_GOES_HERE
  Logical1 : xbsIndex_r4/Logical  logical_function=AND  inputs=2  en=off  latency=0  precision=Full  arith_type=Unsigned  n_bits=8  bin_pt=2  align_bp=on  dbl_ovrd=off  block_type=logical
      settings: xl_area=[1 0 0 1 0 0 0]  block_version=VER_STRING_GOES_HERE
  Q : Outport
  wires:
  Delay/1 -> Inverter/1
  Inverter/1 -> Logical1/1
  Logical1/1 -> Q/1
  D/1 -> Delay/1, Logical1/2

== system wlan_mac_hw/Registers/Sim Start2 ==
  Disregard Subsystem : xbsIndex_r4/Disregard Subsystem  Tag=discardX  block_type=disregard
  Pulse Generator : DiscretePulseGenerator  Period=1e6  PulseWidth=25  PhaseDelay=4e3
  Pulse Generator1 : DiscretePulseGenerator  Period=1e6  PulseWidth=2  PhaseDelay=2.5e4
  sim_only_start : xbsIndex_r4/Gateway In  gui_display_data_type=Boolean  arith_type=Boolean  n_bits=32  bin_pt=0  preci_type=Single  exp_width=8  frac_width=24  quantization="Round  (unbiased: +/- Inf)"  overflow=Saturate  period=1  dbl_ovrd=off  timing_constraint=None  locs_specified=off  LOCs={}  UseAsADC=off  ADCChannel='1'  inherit_from_input=off  hdl_port=on  block_type=gatewayin
  Out1 : Outport
  wires:
  Pulse Generator1/1 -> ?
  Pulse Generator/1 -> sim_only_start/1
  sim_only_start/1 -> Out1/1

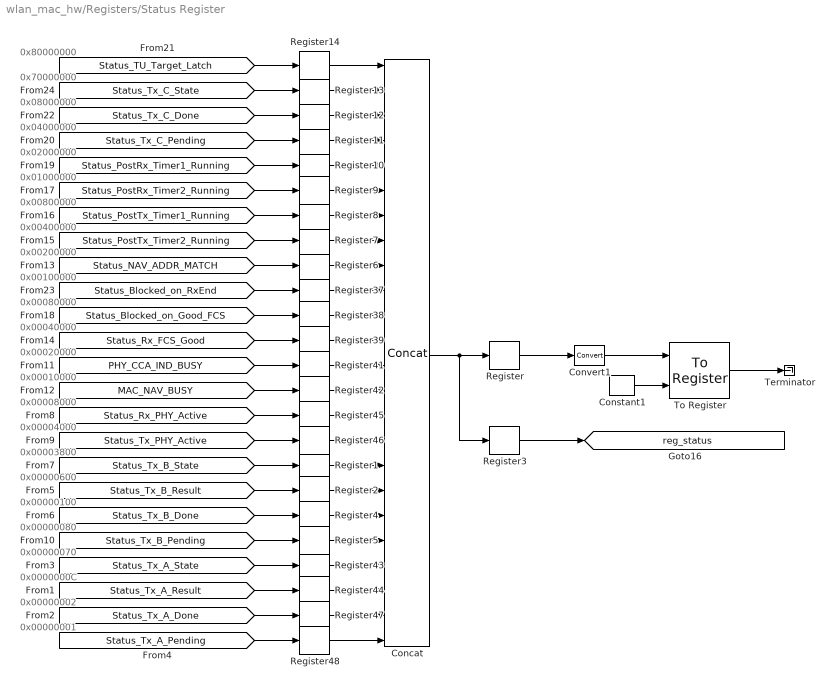
== system wlan_mac_hw/Registers/Status Register ==
  note: 0x00100000
  note: 0x00080000
  note: 0x00040000
  note: 0x00020000
  note: 0x00010000
  note: 0x00008000
  note: 0x00004000
  note: 0x00003800
  note: 0x00000600
  note: 0x00000100
  note: 0x00000080
  note: 0x00000070
  note: 0x0000000C
  note: 0x00000002
  note: 0x00000001
  note: 0x00200000
  note: 0x01000000
  note: 0x00800000
  note: 0x00400000
  note: 0x02000000
  note: 0x04000000
  note: 0x08000000
  note: 0x70000000
  note: 0x80000000
  Concat : xbsIndex_r4/Concat  num_inputs=24  dbl_ovrd=off  block_type=concat
      settings: block_version=8.2.02
  Constant1 : xbsIndex_r4/Constant  const=1  gui_display_data_type=Boolean  arith_type=Boolean  n_bits=30  bin_pt=0  preci_type=Single  exp_width=8  frac_width=24  explicit_period=on  period=1  equ=P=C  opselect=C  inp2=PCIN>>17  opr=+  inp1=P  carry=CIN  dbl_ovrd=off  block_type=constant
  Convert1 : xbsIndex_r4/Convert  gui_display_data_type=Fixed-point  arith_type=Unsigned  n_bits=32  bin_pt=0  float_type=Single  exp_bits=8  fraction_bits=24  quantization=Truncate  overflow=Wrap  en=off  latency=0  dbl_ovrd=off  pipeline=off  block_type=convert
  Register{,1..14,37..39,41..48} (26 alike) : xbsIndex_r4/Register  init=0  rst=off  en=off  dbl_ovrd=off  block_type=register
  Terminator : Terminator
  To Register : xbsIndex_r4/To Register  shared_memory_name='Status'  init=0  ownership=Locally owned and initialized  explicit_data_type=on  gui_display_data_type=Fixed-point  arith_type=Unsigned  n_bits=32  bin_pt=0  preci_type=Single  dbl_ovrd=off  block_type=toreg
      settings: AttributesFormatString=<< %<shared_memory_name> >>  infoedit="Register block that writes data to a shared memory register.  Delay of one sample period."
  tag scope: reg_status=global
  wires:
  Constant1/1 -> To Register/2
  To Register/1 -> Terminator/1
  Register/1 -> Convert1/1
  Convert1/1 -> To Register/1
  Register3/1 -> [reg_status]
  [PHY_CCA_IND_BUSY] -> Register41/1
  [MAC_NAV_BUSY] -> Register42/1
  [Status_Tx_A_State] -> Register43/1
  [Status_Tx_A_Result] -> Register44/1
  [Status_Rx_PHY_Active] -> Register45/1
  [Status_Tx_PHY_Active] -> Register46/1
  [Status_Tx_A_Done] -> Register47/1
  [Status_Tx_A_Pending] -> Register48/1
  [Status_Rx_FCS_Good] -> Register39/1
  [Status_Blocked_on_Good_FCS] -> Register38/1
  [Status_Blocked_on_RxEnd] -> Register37/1
  [Status_Tx_B_State] -> Register1/1
  [Status_Tx_B_Result] -> Register2/1
  [Status_Tx_B_Done] -> Register4/1
  [Status_Tx_B_Pending] -> Register5/1
  [Status_NAV_ADDR_MATCH] -> Register6/1
  Register10/1 -> Concat/5
  Register9/1 -> Concat/6
  Register8/1 -> Concat/7
  Register7/1 -> Concat/8
  Register6/1 -> Concat/9
  Register37/1 -> Concat/10
  Register38/1 -> Concat/11
  Register39/1 -> Concat/12
  Register41/1 -> Concat/13
  Register42/1 -> Concat/14
  Register45/1 -> Concat/15
  Register46/1 -> Concat/16
  Register1/1 -> Concat/17
  Register2/1 -> Concat/18
  Register4/1 -> Concat/19
  Register5/1 -> Concat/20
  Register43/1 -> Concat/21
  Register44/1 -> Concat/22
  Register47/1 -> Concat/23
  Register48/1 -> Concat/24
  [Status_PostRx_Timer1_Running] -> Register10/1
  [Status_PostRx_Timer2_Running] -> Register9/1
  [Status_PostTx_Timer1_Running] -> Register8/1
  [Status_PostTx_Timer2_Running] -> Register7/1
  [Status_Tx_C_State] -> Register13/1
  [Status_Tx_C_Done] -> Register12/1
  [Status_Tx_C_Pending] -> Register11/1
  Register11/1 -> Concat/4
  Register12/1 -> Concat/3
  Register13/1 -> Concat/2
  Concat/1 -> Register/1, Register3/1
  [Status_TU_Target_Latch] -> Register14/1
  Register14/1 -> Concat/1
